simulink model "mophongpid_dienap"  (Simulink 9.0)
settings: Solver=FixedStepAuto  StartTime=0.0  StopTime=10  FixedStep=0.01  RelTol=1e-3
values from neighbouring files (symbols this model uses):
  k = 150    [Bai3.m]    (also in LQR.m = lqr(A,B,Q,R))
  theta_init = 0.1    [LQR.m]
  thetadot_init = 0    [LQR.m]
  x_init = 0    [LQR.m]
  xdot_init = 0    [LQR.m]
settings Model: Creator=ADMIN  LastModifiedBy=ADMIN
settings DataIOCC: SaveFormat=Dataset
settings OptimizationCC: LifeSpan=auto
settings DebuggingCC: UnderspecifiedInitializationDetection=Simplified  MergeDetectMultiDrivingBlocksExec=error  SFUnexpectedBacktrackingDiag=error  SFNoUnconditionalDefaultTransitionDiag=error  SFExecutionAtInitializationDiag=warning
settings HardwareCC: ProdBitPerPointer=64  ProdBitPerSizeT=64  ProdBitPerPtrDiffT=64  ProdLargestAtomicFloat=Float  ProdIntDivRoundTo=Zero  ProdEndianess=LittleEndian  ProdWordSize=64  ProdHWDeviceType=Intel->x86-64 (Windows64)
settings ModelReferenceCC: PropagateSignalLabelsOutOfModel=on
settings CodeAppCC: StateflowObjectComments=off
settings GRTTargetCC: TargetLangStandard=C99 (ISO)
settings ConfigComp: CovMetricSettings=dwe  CovHtmlReporting=off  CovSaveCumulativeToWorkspaceVar=off  CovSaveSingleToWorkspaceVar=off  CovExternalEMLEnable=on

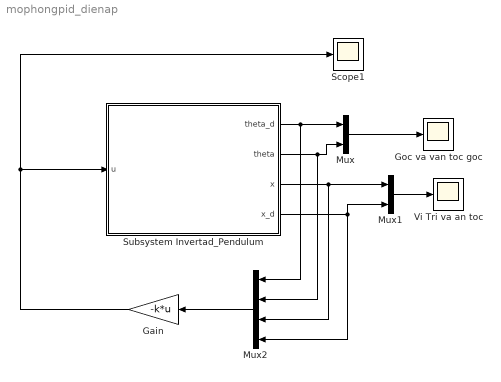
== system mophongpid_dienap ==
  Gain : Gain  Gain=-k*u
  Goc va van toc goc : Scope
  Mux : Mux  Inputs=2
  Mux1 : Mux  Inputs=2
  Mux2 : Mux
  Scope1 : Scope
  Subsystem Invertad_Pendulum : Subsystem
  Vi Tri va an toc : Scope
  wires:
  Subsystem Invertad_Pendulum/1(theta_d) -> Mux2/1, Mux/1
  Subsystem Invertad_Pendulum/2(theta) -> Mux2/2, Mux/2
  Mux/1 -> Goc va van toc goc/1
  Subsystem Invertad_Pendulum/3(x) -> Mux2/3, Mux1/1
  Subsystem Invertad_Pendulum/4(x_d) -> Mux2/4, Mux1/2
  Mux1/1 -> Vi Tri va an toc/1
  Mux2/1 -> Gain/1
  Gain/1 -> Scope1/1, Subsystem Invertad_Pendulum/1(u)

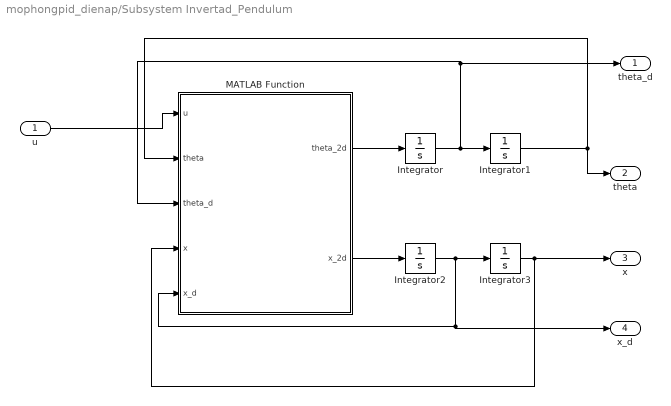
== system mophongpid_dienap/Subsystem Invertad_Pendulum ==
  u : Inport
  Integrator : Integrator  InitialCondition=thetadot_init
  Integrator1 : Integrator  InitialCondition=theta_init
  Integrator2 : Integrator  InitialCondition=xdot_init
  Integrator3 : Integrator  InitialCondition=x_init
  MATLAB Function : MATLAB Function  TreatAsAtomicUnit=on
  theta_d : Outport
  theta : Outport  Port=2
  x : Outport  Port=3
  x_d : Outport  Port=4
  wires:
  MATLAB Function/2(x_2d) -> Integrator2/1
  MATLAB Function/1(theta_2d) -> Integrator/1
  Integrator/1 -> MATLAB Function/3(theta_d), theta_d/1, Integrator1/1
  Integrator2/1 -> MATLAB Function/5(x_d), x_d/1, Integrator3/1
  Integrator3/1 -> MATLAB Function/4(x), x/1
  Integrator1/1 -> theta/1, MATLAB Function/2(theta)
  u/1 -> MATLAB Function/1(u)

== matlab function Subsystem Invertad_Pendulum/MATLAB Function ==
  data: u input double; theta input double; theta_2d output double; theta_d input double; x_2d output double; x input double; x_d input double
function [theta_2d,x_2d] = Inverted_Pendulum(u,theta,theta_d,x,x_d)
M=1;
m=0.1;
l=1;
g=9.81;
x_2d=(u+m*1*sin(theta)*(theta_d)^2-m*g*cos(theta)*sin(theta))/(M+m-m*(cos(theta))^2);
theta_2d =((u*cos(theta)-(M+m)*g*(sin(theta)+m*l*(cos(theta)*sin(theta))*theta_d^2))/(m*l*(cos(theta))^2-(M+m)*l);
